simulink library "Ramp_Library_R2017b"  (R2017b)
settings: Solver=VariableStepAuto  StartTime=0.0  StopTime=10.0  RelTol=1e-3
libraries: simulink x52
(part 2 of 2)

== system Ramp_Library_R2017b/GammaRampLibraryTwoWaysSingleLed/If Action Subsystem ==
  In1 : Inport
  In2 : Inport  Port=2
  Action Port : ActionPort
  Add : Sum  OutDataTypeStr=Inherit: Inherit via back propagation
  Out1 : Outport
  wires:
  In2/1 -> Add/2
  In1/1 -> Add/1
  Add/1 -> Out1/1

== system Ramp_Library_R2017b/GammaRampLibraryTwoWaysSingleLed/If Action Subsystem1 ==
  In1 : Inport
  Action Port : ActionPort
  Out1 : Outport
  wires:
  In1/1 -> Out1/1

== system Ramp_Library_R2017b/GammaRampLibraryTwoWaysSingleLed/If Action Subsystem3 ==
  In1 : Inport
  In2 : Inport  Port=2
  Action Port : ActionPort
  Add : Sum  Inputs=+-  OutDataTypeStr=Inherit: Inherit via back propagation
  Out1 : Outport
  wires:
  In2/1 -> Add/2
  In1/1 -> Add/1
  Add/1 -> Out1/1

== system Ramp_Library_R2017b/GammaRampLibraryTwoWaysSingleLed/RampDownSlopeCalc ==
  V_RampTime100To0 : Inport
  V_SampleTime : Inport  Port=2
  V_DisableRamp : Inport  Port=3
  Enable : EnablePort
  Compare To Zero : simulink/Logic and Bit Operations/Compare To Zero  relop=~=  OutDataTypeStr=boolean
  Constant : Constant  Value=100  OutMin=0  OutMax=100  OutDataTypeStr=fixdt(0,16,0.01,0)
  If : If  IfExpression=u1 ~= 0
  If Action Subsystem : Subsystem  TreatAsAtomicUnit=on
  If Action Subsystem1 : Subsystem  TreatAsAtomicUnit=on
  Logical Operator : Logic  AllPortsSameDT=off  OutDataTypeStr=boolean
  Logical Operator1 : Logic  Operator=NOT  AllPortsSameDT=off  OutDataTypeStr=boolean
  Merge : Merge  InitialOutput=100
  V_RampDownSlope : Outport
  wires:
  If/1 -> If Action Subsystem/Action
  V_RampTime100To0/1 -> If Action Subsystem/2(Denominator), Compare To Zero/1
  Constant/1 -> If Action Subsystem1/1(DefaultValue)
  Merge/1 -> V_RampDownSlope/1
  If Action Subsystem/1(Result) -> Merge/1
  If Action Subsystem1/1(Result) -> Merge/2
  If/2 -> If Action Subsystem1/Action
  V_SampleTime/1 -> If Action Subsystem/1(Numerator)
  Compare To Zero/1 -> Logical Operator/1
  Logical Operator/1 -> If/1
  V_DisableRamp/1 -> Logical Operator1/1
  Logical Operator1/1 -> Logical Operator/2

== system Ramp_Library_R2017b/GammaRampLibraryTwoWaysSingleLed/RampUpSlopeCalc ==
  V_RampTime0To100 : Inport
  V_SampleTime : Inport  Port=2
  V_DisableRamp : Inport  Port=3
  Enable : EnablePort
  Compare To Zero : simulink/Logic and Bit Operations/Compare To Zero  relop=~=  OutDataTypeStr=boolean
  Constant : Constant  Value=100  OutMin=0  OutMax=100  OutDataTypeStr=fixdt(0,16,0.01,0)
  If : If  IfExpression=u1 ~= 0
  If Action Subsystem : Subsystem  TreatAsAtomicUnit=on
  If Action Subsystem1 : Subsystem  TreatAsAtomicUnit=on
  Logical Operator : Logic  AllPortsSameDT=off  OutDataTypeStr=boolean
  Logical Operator1 : Logic  Operator=NOT  AllPortsSameDT=off  OutDataTypeStr=boolean
  Merge : Merge  InitialOutput=100
  V_RampUpSlope : Outport
  wires:
  Logical Operator1/1 -> Logical Operator/2
  V_DisableRamp/1 -> Logical Operator1/1
  Logical Operator/1 -> If/1
  Compare To Zero/1 -> Logical Operator/1
  V_SampleTime/1 -> If Action Subsystem/1(Numerator)
  If/2 -> If Action Subsystem1/Action
  If Action Subsystem1/1(Result) -> Merge/2
  If Action Subsystem/1(Result) -> Merge/1
  Merge/1 -> V_RampUpSlope/1
  Constant/1 -> If Action Subsystem1/1(DefaultValue)
  V_RampTime0To100/1 -> Compare To Zero/1, If Action Subsystem/2(Denominator)
  If/1 -> If Action Subsystem/Action

== system Ramp_Library_R2017b/RampLibraryPwm/Subsystem ==
  LastPWM : Inport
  Action Port : ActionPort
  NewPWM : Outport
  wires:
  LastPWM/1 -> NewPWM/1

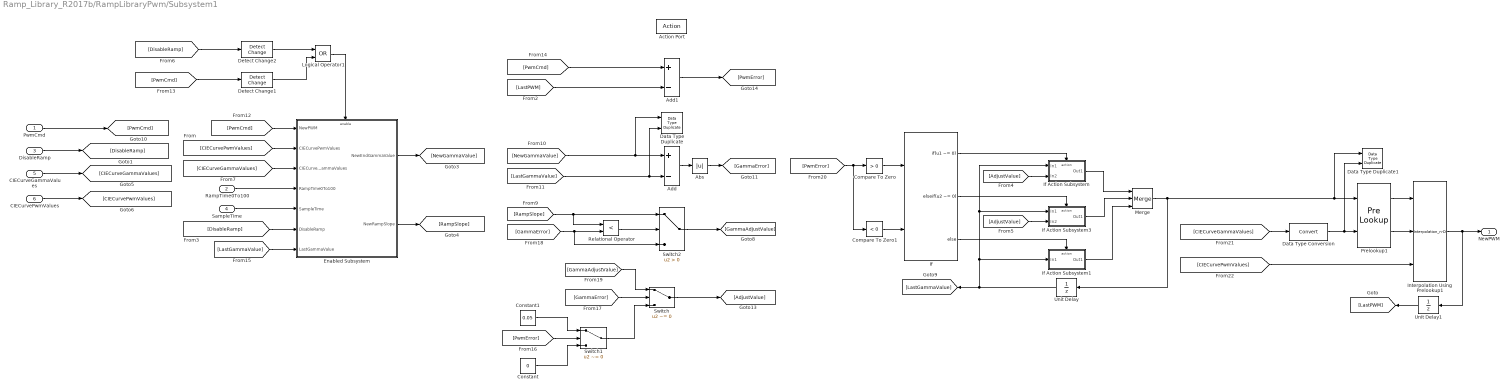
== system Ramp_Library_R2017b/RampLibraryPwm/Subsystem1 ==
  PwmCmd : Inport
  RampTime0To100 : Inport  Port=2
  DisableRamp : Inport  Port=3
  SampleTime : Inport  Port=4
  CIECurveGammaValues : Inport  Port=5
  CIECurvePwmValues : Inport  Port=6
  Action Port : ActionPort
  Abs : Abs  OutDataTypeStr=Inherit: Inherit via internal rule
  Add : Sum  Inputs=+-  OutDataTypeStr=fixdt(1,32,24)
  Add1 : Sum  Inputs=+-  OutDataTypeStr=fixdt(1,16,0.1,0)
  Compare To Zero : simulink/Logic and Bit Operations/Compare To Zero  relop=>  OutDataTypeStr=boolean
  Compare To Zero1 : simulink/Logic and Bit Operations/Compare To Zero  relop=<  OutDataTypeStr=boolean
  Constant : Constant  Value=0  OutDataTypeStr=Inherit: Inherit via back propagation
  Constant1 : Constant  Value=0.05  OutDataTypeStr=Inherit: Inherit via back propagation
  Data Type Duplicate : DataTypeDuplicate
  Data Type Duplicate1 : DataTypeDuplicate
  Data Type Conversion : DataTypeConversion
  Detect Change1 : simulink/Logic and Bit Operations/Detect Change  vinit=0  OutDataTypeStr=boolean
  Detect Change2 : simulink/Logic and Bit Operations/Detect Change  vinit=0  OutDataTypeStr=boolean
  Enabled Subsystem : Subsystem  TreatAsAtomicUnit=on
  If : If  NumInputs=2  IfExpression=u1 ~= 0  ElseIfExpressions=u2 ~= 0
  If Action Subsystem : Subsystem  TreatAsAtomicUnit=on
  If Action Subsystem1 : Subsystem  TreatAsAtomicUnit=on
  If Action Subsystem3 : Subsystem  TreatAsAtomicUnit=on
  Interpolation Using Prelookup1 : Interpolation_n-D  NumberOfTableDimensions=1  TableSource=Input port  ExtrapMethod=Clip  RemoveProtectionIndex=on  ValidIndexMayReachLast=on  InternalRulePriority=Speed  RndMeth=Nearest
      settings: InputPortMap=u0,u1,p2
  Logical Operator1 : Logic  Operator=OR  AllPortsSameDT=off  OutDataTypeStr=boolean
  Merge : Merge  Inputs=3
  Prelookup1 : PreLookup  BreakpointsDataSource=Input port  BreakpointsData=[10:10:110]  BeginIndexSearchUsingPreviousIndexResult=on  UseLastBreakpoint=on  RemoveProtectionInput=on
      settings: InputPortMap=u0,p1
  Relational Operator : RelationalOperator  Operator=<  OutDataTypeStr=boolean  RndMeth=Simplest
  Switch : Switch  Criteria=u2 ~= 0
  Switch1 : Switch  Criteria=u2 ~= 0
  Switch2 : Switch  Criteria=u2 > Threshold  OutDataTypeStr=Inherit: Inherit via back propagation
  Unit Delay : UnitDelay  SampleTime=-1
  Unit Delay1 : UnitDelay  SampleTime=-1
  NewPWM : Outport
  wires:
  [PwmError] -> Compare To Zero/1, Compare To Zero1/1
  Add1/1 -> [PwmError]
  [LastGammaValue] -> Enabled Subsystem/7(LastGammaValue)
  [PwmCmd] -> Detect Change1/1
  [PwmCmd] -> Enabled Subsystem/1(NewPWM)
  PwmCmd/1 -> [PwmCmd]
  [LastGammaValue] -> Add/2, Data Type Duplicate/2
  [NewGammaValue] -> Add/1, Data Type Duplicate/1
  Enabled Subsystem/1(NewEndGammaValue) -> [NewGammaValue]
  Merge/1 -> Prelookup1/1, Data Type Duplicate1/1, Unit Delay/1
  Compare To Zero/1 -> If/1
  SampleTime/1 -> Enabled Subsystem/5(SampleTime)
  Switch2/1 -> [GammaAdjustValue]
  Interpolation Using Prelookup1/1 -> Unit Delay1/1, NewPWM/1
  If/1 -> If Action Subsystem/Action
  Relational Operator/1 -> Switch2/2
  If Action Subsystem1/1(Out1) -> Merge/3
  If Action Subsystem3/1(Out1) -> Merge/2
  If/3 -> If Action Subsystem1/Action
  If Action Subsystem/1(Out1) -> Merge/1
  [AdjustValue] -> If Action Subsystem3/2(In2)
  [AdjustValue] -> If Action Subsystem/2(In2)
  [CIECurvePwmValues] -> Interpolation Using Prelookup1/3
  If/2 -> If Action Subsystem3/Action
  [RampSlope] -> Switch2/1, Relational Operator/1
  Prelookup1/2 -> Interpolation Using Prelookup1/2
  Prelookup1/1 -> Interpolation Using Prelookup1/1
  Compare To Zero1/1 -> If/2
  RampTime0To100/1 -> Enabled Subsystem/4(RampTime0To100)
  Unit Delay/1 -> If Action Subsystem1/1(In1), If Action Subsystem3/1(In1), If Action Subsystem/1(In1), [LastGammaValue]
  Enabled Subsystem/2(NewRampSlope) -> [RampSlope]
  Detect Change2/1 -> Logical Operator1/1
  Detect Change1/1 -> Logical Operator1/2
  DisableRamp/1 -> [DisableRamp]
  [DisableRamp] -> Enabled Subsystem/6(DisableRamp)
  [DisableRamp] -> Detect Change2/1
  Logical Operator1/1 -> Enabled Subsystem/Enable
  Data Type Conversion/1 -> Prelookup1/2, Data Type Duplicate1/2
  [CIECurveGammaValues] -> Data Type Conversion/1
  Add/1 -> Abs/1
  Unit Delay1/1 -> [LastPWM]
  [PwmCmd] -> Add1/1
  [LastPWM] -> Add1/2
  Abs/1 -> [GammaError]
  [GammaError] -> Switch/2
  [GammaError] -> Switch2/3, Relational Operator/2
  [GammaAdjustValue] -> Switch/1
  Switch1/1 -> Switch/3
  [PwmError] -> Switch1/2
  Constant/1 -> Switch1/3
  Constant1/1 -> Switch1/1
  Switch/1 -> [AdjustValue]
  CIECurvePwmValues/1 -> [CIECurvePwmValues]
  CIECurveGammaValues/1 -> [CIECurveGammaValues]
  [CIECurvePwmValues] -> Enabled Subsystem/2(CIECurvePwmValues)
  [CIECurveGammaValues] -> Enabled Subsystem/3(CIECurveGammaValues)

== system Ramp_Library_R2017b/RampLibraryPwmOptimized/Subsystem ==
  LastPWM : Inport
  Action Port : ActionPort
  NewPWM : Outport
  wires:
  LastPWM/1 -> NewPWM/1

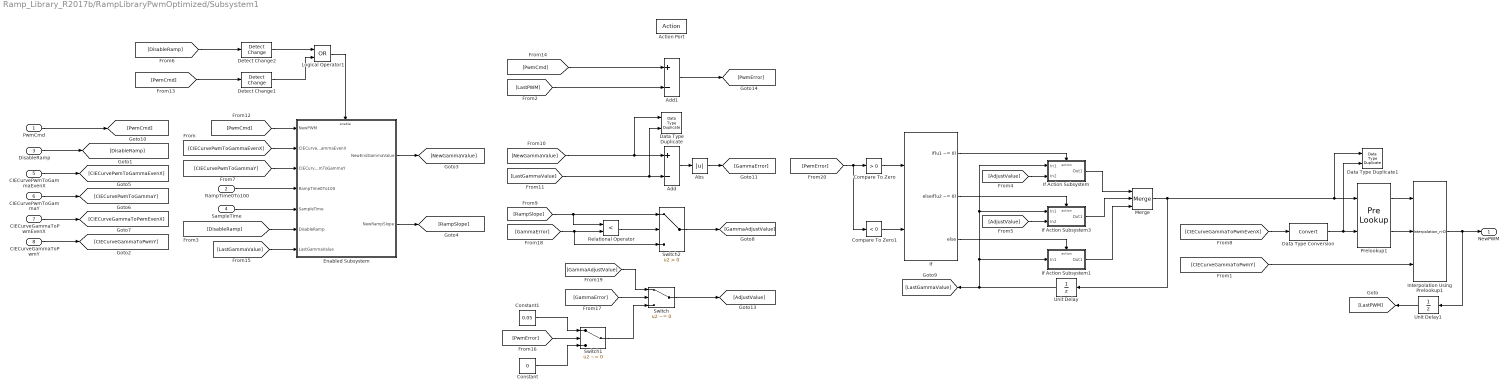
== system Ramp_Library_R2017b/RampLibraryPwmOptimized/Subsystem1 ==
  PwmCmd : Inport
  RampTime0To100 : Inport  Port=2
  DisableRamp : Inport  Port=3
  SampleTime : Inport  Port=4
  CIECurvePwmToGammaEvenX : Inport  Port=5
  CIECurvePwmToGammaY : Inport  Port=6
  CIECurveGammaToPwmEvenX : Inport  Port=7
  CIECurveGammaToPwmY : Inport  Port=8
  Action Port : ActionPort
  Abs : Abs  OutDataTypeStr=Inherit: Inherit via internal rule
  Add : Sum  Inputs=+-  OutDataTypeStr=fixdt(1,32,24)
  Add1 : Sum  Inputs=+-  OutDataTypeStr=fixdt(1,16,0.1,0)
  Compare To Zero : simulink/Logic and Bit Operations/Compare To Zero  relop=>  OutDataTypeStr=boolean
  Compare To Zero1 : simulink/Logic and Bit Operations/Compare To Zero  relop=<  OutDataTypeStr=boolean
  Constant : Constant  Value=0  OutDataTypeStr=Inherit: Inherit via back propagation
  Constant1 : Constant  Value=0.05  OutDataTypeStr=Inherit: Inherit via back propagation
  Data Type Duplicate : DataTypeDuplicate
  Data Type Duplicate1 : DataTypeDuplicate
  Data Type Conversion : DataTypeConversion
  Detect Change1 : simulink/Logic and Bit Operations/Detect Change  vinit=0  OutDataTypeStr=boolean
  Detect Change2 : simulink/Logic and Bit Operations/Detect Change  vinit=0  OutDataTypeStr=boolean
  Enabled Subsystem : Subsystem  TreatAsAtomicUnit=on
  If : If  NumInputs=2  IfExpression=u1 ~= 0  ElseIfExpressions=u2 ~= 0
  If Action Subsystem : Subsystem  TreatAsAtomicUnit=on
  If Action Subsystem1 : Subsystem  TreatAsAtomicUnit=on
  If Action Subsystem3 : Subsystem  TreatAsAtomicUnit=on
  Interpolation Using Prelookup1 : Interpolation_n-D  NumberOfTableDimensions=1  TableSource=Input port  ExtrapMethod=Clip  RemoveProtectionIndex=on  ValidIndexMayReachLast=on  InternalRulePriority=Speed  RndMeth=Nearest
      settings: InputPortMap=u0,u1,p2
  Logical Operator1 : Logic  Operator=OR  AllPortsSameDT=off  OutDataTypeStr=boolean
  Merge : Merge  Inputs=3
  Prelookup1 : PreLookup  BreakpointsDataSource=Input port  BreakpointsData=[10:10:110]  IndexSearchMethod=Evenly spaced points  BeginIndexSearchUsingPreviousIndexResult=on  UseLastBreakpoint=on  RemoveProtectionInput=on
      settings: InputPortMap=u0,p1
  Relational Operator : RelationalOperator  Operator=<  OutDataTypeStr=boolean  RndMeth=Simplest
  Switch : Switch  Criteria=u2 ~= 0
  Switch1 : Switch  Criteria=u2 ~= 0
  Switch2 : Switch  Criteria=u2 > Threshold  OutDataTypeStr=Inherit: Inherit via back propagation
  Unit Delay : UnitDelay  SampleTime=-1
  Unit Delay1 : UnitDelay  SampleTime=-1
  NewPWM : Outport
  wires:
  [PwmError] -> Compare To Zero/1, Compare To Zero1/1
  Add1/1 -> [PwmError]
  [LastGammaValue] -> Enabled Subsystem/7(LastGammaValue)
  [PwmCmd] -> Detect Change1/1
  [PwmCmd] -> Enabled Subsystem/1(NewPWM)
  PwmCmd/1 -> [PwmCmd]
  [LastGammaValue] -> Add/2, Data Type Duplicate/2
  [NewGammaValue] -> Add/1, Data Type Duplicate/1
  Enabled Subsystem/1(NewEndGammaValue) -> [NewGammaValue]
  Merge/1 -> Prelookup1/1, Data Type Duplicate1/1, Unit Delay/1
  Compare To Zero/1 -> If/1
  SampleTime/1 -> Enabled Subsystem/5(SampleTime)
  Switch2/1 -> [GammaAdjustValue]
  Interpolation Using Prelookup1/1 -> Unit Delay1/1, NewPWM/1
  If/1 -> If Action Subsystem/Action
  Relational Operator/1 -> Switch2/2
  If Action Subsystem1/1(Out1) -> Merge/3
  If Action Subsystem3/1(Out1) -> Merge/2
  If/3 -> If Action Subsystem1/Action
  If Action Subsystem/1(Out1) -> Merge/1
  [AdjustValue] -> If Action Subsystem3/2(In2)
  [AdjustValue] -> If Action Subsystem/2(In2)
  [CIECurveGammaToPwmY] -> Interpolation Using Prelookup1/3
  If/2 -> If Action Subsystem3/Action
  [RampSlope] -> Switch2/1, Relational Operator/1
  Prelookup1/2 -> Interpolation Using Prelookup1/2
  Prelookup1/1 -> Interpolation Using Prelookup1/1
  Compare To Zero1/1 -> If/2
  RampTime0To100/1 -> Enabled Subsystem/4(RampTime0To100)
  Unit Delay/1 -> If Action Subsystem1/1(In1), If Action Subsystem3/1(In1), If Action Subsystem/1(In1), [LastGammaValue]
  [CIECurvePwmToGammaEvenX] -> Enabled Subsystem/2(CIECurvePwmToGammaEvenX)
  [CIECurvePwmToGammaY] -> Enabled Subsystem/3(CIECurvePwmToGammaY)
  Enabled Subsystem/2(NewRampSlope) -> [RampSlope]
  Detect Change2/1 -> Logical Operator1/1
  Detect Change1/1 -> Logical Operator1/2
  DisableRamp/1 -> [DisableRamp]
  [DisableRamp] -> Enabled Subsystem/6(DisableRamp)
  [DisableRamp] -> Detect Change2/1
  Logical Operator1/1 -> Enabled Subsystem/Enable
  Data Type Conversion/1 -> Prelookup1/2, Data Type Duplicate1/2
  CIECurvePwmToGammaEvenX/1 -> [CIECurvePwmToGammaEvenX]
  CIECurveGammaToPwmY/1 -> [CIECurveGammaToPwmY]
  CIECurvePwmToGammaY/1 -> [CIECurvePwmToGammaY]
  CIECurveGammaToPwmEvenX/1 -> [CIECurveGammaToPwmEvenX]
  [CIECurveGammaToPwmEvenX] -> Data Type Conversion/1
  Add/1 -> Abs/1
  Unit Delay1/1 -> [LastPWM]
  [PwmCmd] -> Add1/1
  [LastPWM] -> Add1/2
  Abs/1 -> [GammaError]
  [GammaError] -> Switch/2
  [GammaError] -> Switch2/3, Relational Operator/2
  [GammaAdjustValue] -> Switch/1
  Switch1/1 -> Switch/3
  [PwmError] -> Switch1/2
  Constant/1 -> Switch1/3
  Constant1/1 -> Switch1/1
  Switch/1 -> [AdjustValue]

== system Ramp_Library_R2017b/GammaRampLibraryPerLed/RampSlopeCalc/If Action Subsystem ==
  Numerator : Inport
  Denominator : Inport  Port=2
  Action Port : ActionPort
  Divide1 : Product  Inputs=*/  OutDataTypeStr=Inherit: Inherit via back propagation
  Gain1 : Gain  Gain=100  OutDataTypeStr=fixdt(0,32,0.00005,0)
  Result : Outport
  wires:
  Gain1/1 -> Divide1/1
  Denominator/1 -> Divide1/2
  Numerator/1 -> Gain1/1
  Divide1/1 -> Result/1

== system Ramp_Library_R2017b/GammaRampLibraryPerLed/RampSlopeCalc/If Action Subsystem1 ==
  DefaultValue : Inport
  Action Port : ActionPort
  Result : Outport
  wires:
  DefaultValue/1 -> Result/1

== system Ramp_Library_R2017b/GammaRampLibraryPerLedGroup/For Each Subsystem/If Action Subsystem ==
  In1 : Inport
  In2 : Inport  Port=2
  Action Port : ActionPort
  Add : Sum  OutDataTypeStr=Inherit: Inherit via back propagation
  Out1 : Outport
  wires:
  In2/1 -> Add/2
  In1/1 -> Add/1
  Add/1 -> Out1/1

== system Ramp_Library_R2017b/GammaRampLibraryPerLedGroup/For Each Subsystem/If Action Subsystem1 ==
  In1 : Inport
  Action Port : ActionPort
  Out1 : Outport
  wires:
  In1/1 -> Out1/1

== system Ramp_Library_R2017b/GammaRampLibraryPerLedGroup/For Each Subsystem/If Action Subsystem3 ==
  In1 : Inport
  In2 : Inport  Port=2
  Action Port : ActionPort
  Add : Sum  Inputs=+-  OutDataTypeStr=Inherit: Inherit via back propagation
  Out1 : Outport
  wires:
  In2/1 -> Add/2
  In1/1 -> Add/1
  Add/1 -> Out1/1

== system Ramp_Library_R2017b/GammaRampLibraryPerLedGroup/RampSlopeCalc/If Action Subsystem ==
  Numerator : Inport
  Denominator : Inport  Port=2
  Action Port : ActionPort
  Divide1 : Product  Inputs=*/  OutDataTypeStr=Inherit: Inherit via back propagation
  Gain1 : Gain  Gain=100  OutDataTypeStr=fixdt(0,32,0.00005,0)
  Result : Outport
  wires:
  Divide1/1 -> Result/1
  Numerator/1 -> Gain1/1
  Denominator/1 -> Divide1/2
  Gain1/1 -> Divide1/1

== system Ramp_Library_R2017b/GammaRampLibraryPerLedGroup/RampSlopeCalc/If Action Subsystem1 ==
  DefaultValue : Inport
  Action Port : ActionPort
  Result : Outport
  wires:
  DefaultValue/1 -> Result/1

== system Ramp_Library_R2017b/GammaRampLibrarySingleLed/RampSlopeCalc/If Action Subsystem ==
  Numerator : Inport
  Denominator : Inport  Port=2
  Action Port : ActionPort
  Divide1 : Product  Inputs=*/  OutDataTypeStr=Inherit: Inherit via back propagation
  Gain1 : Gain  Gain=100  OutDataTypeStr=fixdt(0,32,0.00005,0)
  Result : Outport
  wires:
  Divide1/1 -> Result/1
  Numerator/1 -> Gain1/1
  Denominator/1 -> Divide1/2
  Gain1/1 -> Divide1/1

== system Ramp_Library_R2017b/GammaRampLibrarySingleLed/RampSlopeCalc/If Action Subsystem1 ==
  DefaultValue : Inport
  Action Port : ActionPort
  Result : Outport
  wires:
  DefaultValue/1 -> Result/1

== system Ramp_Library_R2017b/GammaRampLibraryTwoWaysPerLed/RampDownSlopeCalc/If Action Subsystem ==
  Numerator : Inport
  Denominator : Inport  Port=2
  Action Port : ActionPort
  Divide1 : Product  Inputs=*/  OutDataTypeStr=Inherit: Inherit via back propagation
  Gain1 : Gain  Gain=100  OutDataTypeStr=fixdt(0,32,0.00005,0)
  Result : Outport
  wires:
  Divide1/1 -> Result/1
  Numerator/1 -> Gain1/1
  Denominator/1 -> Divide1/2
  Gain1/1 -> Divide1/1

== system Ramp_Library_R2017b/GammaRampLibraryTwoWaysPerLed/RampDownSlopeCalc/If Action Subsystem1 ==
  DefaultValue : Inport
  Action Port : ActionPort
  Result : Outport
  wires:
  DefaultValue/1 -> Result/1

== system Ramp_Library_R2017b/GammaRampLibraryTwoWaysPerLed/RampUpSlopeCalc/If Action Subsystem ==
  Numerator : Inport
  Denominator : Inport  Port=2
  Action Port : ActionPort
  Divide1 : Product  Inputs=*/  OutDataTypeStr=Inherit: Inherit via back propagation
  Gain1 : Gain  Gain=100  OutDataTypeStr=fixdt(0,32,0.00005,0)
  Result : Outport
  wires:
  Gain1/1 -> Divide1/1
  Denominator/1 -> Divide1/2
  Numerator/1 -> Gain1/1
  Divide1/1 -> Result/1

== system Ramp_Library_R2017b/GammaRampLibraryTwoWaysPerLed/RampUpSlopeCalc/If Action Subsystem1 ==
  DefaultValue : Inport
  Action Port : ActionPort
  Result : Outport
  wires:
  DefaultValue/1 -> Result/1

== system Ramp_Library_R2017b/GammaRampLibraryTwoWaysPerLedGroup/For Each Subsystem/If Action Subsystem ==
  In1 : Inport
  In2 : Inport  Port=2
  Action Port : ActionPort
  Add : Sum  OutDataTypeStr=Inherit: Inherit via back propagation
  Out1 : Outport
  wires:
  Add/1 -> Out1/1
  In1/1 -> Add/1
  In2/1 -> Add/2

== system Ramp_Library_R2017b/GammaRampLibraryTwoWaysPerLedGroup/For Each Subsystem/If Action Subsystem1 ==
  In1 : Inport
  Action Port : ActionPort
  Out1 : Outport
  wires:
  In1/1 -> Out1/1

== system Ramp_Library_R2017b/GammaRampLibraryTwoWaysPerLedGroup/For Each Subsystem/If Action Subsystem3 ==
  In1 : Inport
  In2 : Inport  Port=2
  Action Port : ActionPort
  Add : Sum  Inputs=+-  OutDataTypeStr=Inherit: Inherit via back propagation
  Out1 : Outport
  wires:
  Add/1 -> Out1/1
  In1/1 -> Add/1
  In2/1 -> Add/2

== system Ramp_Library_R2017b/GammaRampLibraryTwoWaysPerLedGroup/RampDownSlopeCalc/If Action Subsystem ==
  Numerator : Inport
  Denominator : Inport  Port=2
  Action Port : ActionPort
  Divide1 : Product  Inputs=*/  OutDataTypeStr=Inherit: Inherit via back propagation
  Gain1 : Gain  Gain=100  OutDataTypeStr=fixdt(0,32,0.00005,0)
  Result : Outport
  wires:
  Divide1/1 -> Result/1
  Numerator/1 -> Gain1/1
  Denominator/1 -> Divide1/2
  Gain1/1 -> Divide1/1

== system Ramp_Library_R2017b/GammaRampLibraryTwoWaysPerLedGroup/RampDownSlopeCalc/If Action Subsystem1 ==
  DefaultValue : Inport
  Action Port : ActionPort
  Result : Outport
  wires:
  DefaultValue/1 -> Result/1

== system Ramp_Library_R2017b/GammaRampLibraryTwoWaysPerLedGroup/RampUpSlopeCalc/If Action Subsystem ==
  Numerator : Inport
  Denominator : Inport  Port=2
  Action Port : ActionPort
  Divide1 : Product  Inputs=*/  OutDataTypeStr=Inherit: Inherit via back propagation
  Gain1 : Gain  Gain=100  OutDataTypeStr=fixdt(0,32,0.00005,0)
  Result : Outport
  wires:
  Gain1/1 -> Divide1/1
  Denominator/1 -> Divide1/2
  Numerator/1 -> Gain1/1
  Divide1/1 -> Result/1

== system Ramp_Library_R2017b/GammaRampLibraryTwoWaysPerLedGroup/RampUpSlopeCalc/If Action Subsystem1 ==
  DefaultValue : Inport
  Action Port : ActionPort
  Result : Outport
  wires:
  DefaultValue/1 -> Result/1

== system Ramp_Library_R2017b/GammaRampLibraryTwoWaysSingleLed/RampDownSlopeCalc/If Action Subsystem ==
  Numerator : Inport
  Denominator : Inport  Port=2
  Action Port : ActionPort
  Divide1 : Product  Inputs=*/  OutDataTypeStr=Inherit: Inherit via back propagation
  Gain1 : Gain  Gain=100  OutDataTypeStr=fixdt(0,32,0.00005,0)
  Result : Outport
  wires:
  Gain1/1 -> Divide1/1
  Denominator/1 -> Divide1/2
  Numerator/1 -> Gain1/1
  Divide1/1 -> Result/1

== system Ramp_Library_R2017b/GammaRampLibraryTwoWaysSingleLed/RampDownSlopeCalc/If Action Subsystem1 ==
  DefaultValue : Inport
  Action Port : ActionPort
  Result : Outport
  wires:
  DefaultValue/1 -> Result/1

== system Ramp_Library_R2017b/GammaRampLibraryTwoWaysSingleLed/RampUpSlopeCalc/If Action Subsystem ==
  Numerator : Inport
  Denominator : Inport  Port=2
  Action Port : ActionPort
  Divide1 : Product  Inputs=*/  OutDataTypeStr=Inherit: Inherit via back propagation
  Gain1 : Gain  Gain=100  OutDataTypeStr=fixdt(0,32,0.00005,0)
  Result : Outport
  wires:
  Divide1/1 -> Result/1
  Numerator/1 -> Gain1/1
  Denominator/1 -> Divide1/2
  Gain1/1 -> Divide1/1

== system Ramp_Library_R2017b/GammaRampLibraryTwoWaysSingleLed/RampUpSlopeCalc/If Action Subsystem1 ==
  DefaultValue : Inport
  Action Port : ActionPort
  Result : Outport
  wires:
  DefaultValue/1 -> Result/1

== system Ramp_Library_R2017b/RampLibraryPwm/Subsystem1/Enabled Subsystem ==
  NewPWM : Inport
  CIECurvePwmValues : Inport  Port=2
  CIECurveGammaValues : Inport  Port=3
  RampTime0To100 : Inport  Port=4
  SampleTime : Inport  Port=5
  DisableRamp : Inport  Port=6
  LastGammaValue : Inport  Port=7
  Enable : EnablePort
  Abs : Abs  OutDataTypeStr=Inherit: Inherit via internal rule
  Abs1 : Abs  OutDataTypeStr=Inherit: Inherit via internal rule
  Constant : Constant  Value=100  OutDataTypeStr=uint8
  Constant1 : Constant  Value=100  OutDataTypeStr=fixdt(0,32,24)
  Data Type Duplicate : DataTypeDuplicate
  Data Type Conversion1 : DataTypeConversion
  Divide : Product  Inputs=**//  OutDataTypeStr=fixdt(0,32,0.005,0)
  Interpolation Using Prelookup : Interpolation_n-D  NumberOfTableDimensions=1  TableSource=Input port  ExtrapMethod=Clip  RemoveProtectionIndex=on  ValidIndexMayReachLast=on  OutMin=0  OutMax=100  OutDataTypeStr=fixdt(0,32,24)  InternalRulePriority=Speed
      settings: InputPortMap=u0,u1,p2
  Prelookup : PreLookup  BreakpointsDataSource=Input port  BreakpointsData=[10:10:110]  BeginIndexSearchUsingPreviousIndexResult=on  UseLastBreakpoint=on  RemoveProtectionInput=on
      settings: InputPortMap=u0,p1
  SimpleSecureDivision : Subsystem
  Subtract : Sum  Inputs=+-  OutDataTypeStr=fixdt(1,32,24)
  Subtract1 : Sum  Inputs=+-  OutDataTypeStr=fixdt(1,16,0.1,0)
  Switch : Switch  Criteria=u2 ~= 0
  Unit Delay : UnitDelay  SampleTime=-1
  NewEndGammaValue : Outport
  NewRampSlope : Outport  Port=2
  wires:
  Prelookup/2 -> Interpolation Using Prelookup/2
  Prelookup/1 -> Interpolation Using Prelookup/1
  Data Type Conversion1/1 -> Data Type Duplicate/2, Prelookup/2
  Interpolation Using Prelookup/1 -> Subtract/1, NewEndGammaValue/1
  NewPWM/1 -> Data Type Duplicate/1, Prelookup/1, Subtract1/1, Unit Delay/1
  CIECurvePwmValues/1 -> Data Type Conversion1/1
  CIECurveGammaValues/1 -> Interpolation Using Prelookup/3
  RampTime0To100/1 -> Divide/2
  Constant/1 -> Divide/3
  LastGammaValue/1 -> Subtract/2
  Subtract/1 -> Abs/1
  Divide/1 -> SimpleSecureDivision/2(Denominator)
  SampleTime/1 -> Divide/4
  Abs/1 -> Switch/1, SimpleSecureDivision/1(Numerator)
  DisableRamp/1 -> [DisableRamp]
  SimpleSecureDivision/1(Result) -> Switch/3
  Switch/1 -> NewRampSlope/1
  [DisableRamp] -> Switch/2
  Subtract1/1 -> Abs1/1
  Unit Delay/1 -> Subtract1/2
  Abs1/1 -> Divide/1
  Constant1/1 -> SimpleSecureDivision/3(DefaultValue)

== system Ramp_Library_R2017b/RampLibraryPwm/Subsystem1/If Action Subsystem ==
  In1 : Inport
  In2 : Inport  Port=2
  Action Port : ActionPort
  Add : Sum  OutDataTypeStr=Inherit: Inherit via back propagation
  Out1 : Outport
  wires:
  Add/1 -> Out1/1
  In2/1 -> Add/2
  In1/1 -> Add/1

== system Ramp_Library_R2017b/RampLibraryPwm/Subsystem1/If Action Subsystem1 ==
  In1 : Inport
  Action Port : ActionPort
  Out1 : Outport
  wires:
  In1/1 -> Out1/1

== system Ramp_Library_R2017b/RampLibraryPwm/Subsystem1/If Action Subsystem3 ==
  In1 : Inport
  In2 : Inport  Port=2
  Action Port : ActionPort
  Add : Sum  Inputs=+-  OutDataTypeStr=Inherit: Inherit via back propagation
  Out1 : Outport
  wires:
  Add/1 -> Out1/1
  In2/1 -> Add/2
  In1/1 -> Add/1

== system Ramp_Library_R2017b/RampLibraryPwmOptimized/Subsystem1/Enabled Subsystem ==
  NewPWM : Inport
  CIECurvePwmToGammaEvenX : Inport  Port=2
  CIECurvePwmToGammaY : Inport  Port=3
  RampTime0To100 : Inport  Port=4
  SampleTime : Inport  Port=5
  DisableRamp : Inport  Port=6
  LastGammaValue : Inport  Port=7
  Enable : EnablePort
  Abs : Abs  OutDataTypeStr=Inherit: Inherit via internal rule
  Abs1 : Abs  OutDataTypeStr=Inherit: Inherit via internal rule
  Constant : Constant  Value=100  OutDataTypeStr=uint8
  Constant1 : Constant  Value=100  OutDataTypeStr=fixdt(0,32,24)
  Data Type Duplicate : DataTypeDuplicate
  Data Type Conversion1 : DataTypeConversion
  Divide : Product  Inputs=**//  OutDataTypeStr=fixdt(0,32,0.005,0)
  Interpolation Using Prelookup : Interpolation_n-D  NumberOfTableDimensions=1  TableSource=Input port  ExtrapMethod=Clip  RemoveProtectionIndex=on  ValidIndexMayReachLast=on  OutMin=0  OutMax=100  OutDataTypeStr=fixdt(0,32,24)  InternalRulePriority=Speed
      settings: InputPortMap=u0,u1,p2
  Prelookup : PreLookup  BreakpointsDataSource=Input port  BreakpointsData=[10:10:110]  IndexSearchMethod=Evenly spaced points  BeginIndexSearchUsingPreviousIndexResult=on  UseLastBreakpoint=on  RemoveProtectionInput=on
      settings: InputPortMap=u0,p1
  SimpleSecureDivision : Subsystem
  Subtract : Sum  Inputs=+-  OutDataTypeStr=fixdt(1,32,24)
  Subtract1 : Sum  Inputs=+-  OutDataTypeStr=fixdt(1,16,0.1,0)
  Switch : Switch  Criteria=u2 ~= 0
  Unit Delay : UnitDelay  SampleTime=-1
  NewEndGammaValue : Outport
  NewRampSlope : Outport  Port=2
  wires:
  Prelookup/2 -> Interpolation Using Prelookup/2
  Prelookup/1 -> Interpolation Using Prelookup/1
  Data Type Conversion1/1 -> Data Type Duplicate/2, Prelookup/2
  Interpolation Using Prelookup/1 -> Subtract/1, NewEndGammaValue/1
  NewPWM/1 -> Data Type Duplicate/1, Prelookup/1, Subtract1/1, Unit Delay/1
  CIECurvePwmToGammaEvenX/1 -> Data Type Conversion1/1
  CIECurvePwmToGammaY/1 -> Interpolation Using Prelookup/3
  RampTime0To100/1 -> Divide/2
  Constant/1 -> Divide/3
  LastGammaValue/1 -> Subtract/2
  Subtract/1 -> Abs/1
  Divide/1 -> SimpleSecureDivision/2(Denominator)
  SampleTime/1 -> Divide/4
  Abs/1 -> Switch/1, SimpleSecureDivision/1(Numerator)
  DisableRamp/1 -> [DisableRamp]
  SimpleSecureDivision/1(Result) -> Switch/3
  Switch/1 -> NewRampSlope/1
  [DisableRamp] -> Switch/2
  Subtract1/1 -> Abs1/1
  Unit Delay/1 -> Subtract1/2
  Abs1/1 -> Divide/1
  Constant1/1 -> SimpleSecureDivision/3(DefaultValue)

== system Ramp_Library_R2017b/RampLibraryPwmOptimized/Subsystem1/If Action Subsystem ==
  In1 : Inport
  In2 : Inport  Port=2
  Action Port : ActionPort
  Add : Sum  OutDataTypeStr=Inherit: Inherit via back propagation
  Out1 : Outport
  wires:
  Add/1 -> Out1/1
  In2/1 -> Add/2
  In1/1 -> Add/1

== system Ramp_Library_R2017b/RampLibraryPwmOptimized/Subsystem1/If Action Subsystem1 ==
  In1 : Inport
  Action Port : ActionPort
  Out1 : Outport
  wires:
  In1/1 -> Out1/1

== system Ramp_Library_R2017b/RampLibraryPwmOptimized/Subsystem1/If Action Subsystem3 ==
  In1 : Inport
  In2 : Inport  Port=2
  Action Port : ActionPort
  Add : Sum  Inputs=+-  OutDataTypeStr=Inherit: Inherit via back propagation
  Out1 : Outport
  wires:
  Add/1 -> Out1/1
  In2/1 -> Add/2
  In1/1 -> Add/1

== system Ramp_Library_R2017b/RampLibraryPwm/Subsystem1/Enabled Subsystem/SimpleSecureDivision ==
  Numerator : Inport
  Denominator : Inport  Port=2
  DefaultValue : Inport  Port=3
  Compare To Zero : simulink/Logic and Bit Operations/Compare To Zero  relop=~=  OutDataTypeStr=boolean
  If : If  IfExpression=u1 ~= 0
  If Action Subsystem : Subsystem  TreatAsAtomicUnit=on
  If Action Subsystem1 : Subsystem  TreatAsAtomicUnit=on
  Merge : Merge  InitialOutput=100
  Result : Outport
  wires:
  Numerator/1 -> If Action Subsystem/1(Numerator)
  If/2 -> If Action Subsystem1/Action
  Denominator/1 -> If Action Subsystem/2(Denominator), Compare To Zero/1
  If Action Subsystem/1(Result) -> Merge/1
  If Action Subsystem1/1(Result) -> Merge/2
  Merge/1 -> Result/1
  DefaultValue/1 -> If Action Subsystem1/1(DefaultValue)
  If/1 -> If Action Subsystem/Action
  Compare To Zero/1 -> If/1

== system Ramp_Library_R2017b/RampLibraryPwmOptimized/Subsystem1/Enabled Subsystem/SimpleSecureDivision ==
  Numerator : Inport
  Denominator : Inport  Port=2
  DefaultValue : Inport  Port=3
  Compare To Zero : simulink/Logic and Bit Operations/Compare To Zero  relop=~=  OutDataTypeStr=boolean
  If : If  IfExpression=u1 ~= 0
  If Action Subsystem : Subsystem  TreatAsAtomicUnit=on
  If Action Subsystem1 : Subsystem  TreatAsAtomicUnit=on
  Merge : Merge  InitialOutput=100
  Result : Outport
  wires:
  Numerator/1 -> If Action Subsystem/1(Numerator)
  If/2 -> If Action Subsystem1/Action
  Denominator/1 -> If Action Subsystem/2(Denominator), Compare To Zero/1
  If Action Subsystem/1(Result) -> Merge/1
  If Action Subsystem1/1(Result) -> Merge/2
  Merge/1 -> Result/1
  DefaultValue/1 -> If Action Subsystem1/1(DefaultValue)
  If/1 -> If Action Subsystem/Action
  Compare To Zero/1 -> If/1

== system Ramp_Library_R2017b/RampLibraryPwm/Subsystem1/Enabled Subsystem/SimpleSecureDivision/If Action Subsystem ==
  Numerator : Inport
  Denominator : Inport  Port=2
  Action Port : ActionPort
  Divide : Product  Inputs=*/  OutDataTypeStr=Inherit: Inherit via back propagation
  Result : Outport
  wires:
  Divide/1 -> Result/1
  Numerator/1 -> Divide/1
  Denominator/1 -> Divide/2

== system Ramp_Library_R2017b/RampLibraryPwm/Subsystem1/Enabled Subsystem/SimpleSecureDivision/If Action Subsystem1 ==
  DefaultValue : Inport
  Action Port : ActionPort
  Result : Outport
  wires:
  DefaultValue/1 -> Result/1

== system Ramp_Library_R2017b/RampLibraryPwmOptimized/Subsystem1/Enabled Subsystem/SimpleSecureDivision/If Action Subsystem ==
  Numerator : Inport
  Denominator : Inport  Port=2
  Action Port : ActionPort
  Divide : Product  Inputs=*/  OutDataTypeStr=Inherit: Inherit via back propagation
  Result : Outport
  wires:
  Divide/1 -> Result/1
  Numerator/1 -> Divide/1
  Denominator/1 -> Divide/2

== system Ramp_Library_R2017b/RampLibraryPwmOptimized/Subsystem1/Enabled Subsystem/SimpleSecureDivision/If Action Subsystem1 ==
  DefaultValue : Inport
  Action Port : ActionPort
  Result : Outport
  wires:
  DefaultValue/1 -> Result/1
